simulink model "cccharging"  (R2026a)
settings: Solver=VariableStepAuto  StopTime=3600*nHours
InitFcn:
  | CCCV_parameters
libraries: fl_lib x4, batt_lib x2, nesl_utility x1
settings Model: Creator=clapierr  LastModifiedBy=User
settings SimscapeCC: SimscapeNominalValues="[{\"value\":\"1\",\"unit\":\"A\"},{\"value\":\"1\",\"unit\":\"bar\"},{\"value\":\"1\",\"unit\":\"cm^2\"},{\"value\":\"1\",\"unit\":\"cm^3/s\"},{\"value\":\"1\",\"unit\":\"kJ/kg\"},{\"value\":\"1\",\"unit\":\"kW\"},{\"value\":\"1\",\"unit\":\"l\"},{\"value\":\"1\",\"unit\":\"N\"},{\"value\":\"1\",\"unit\":\"N*m\"},{\"value\":\"1\",\"unit\":\"V\"}]"  SimscapeLogType=none  SimscapeLogDataHistory=5000.0

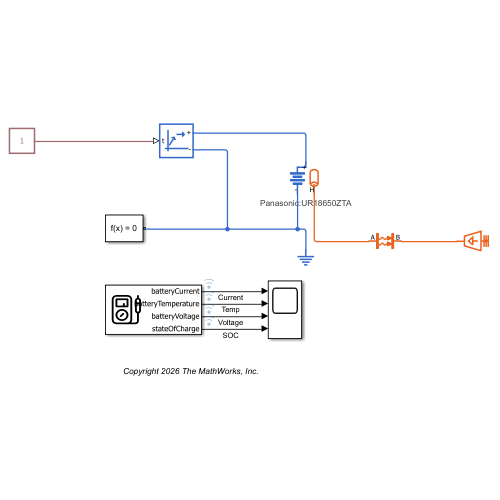
[thumbnail: Simulink's stored preview of the top-level diagram]
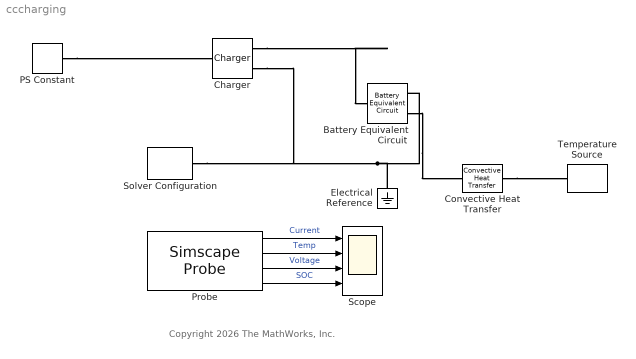
== system cccharging ==
  note: Copyright 2026 The MathWorks, Inc.
  Battery Equivalent Circuit : batt_lib/Cells/Battery Equivalent Circuit  PartSpecification="{\"CollectionId\":\"MW.SimscapeBattery\",\"CollectionVersion\":\"1.0.0\",\"DatasetId\":\"Panasonic|UR18650ZTA|simscape.battery.batteryEquivalentCircuit\",\"DisplayName\":\"Panasonic:UR18650ZTA\"}"  BatteryCapacity=2.65 % Datasheet derived hr*A  ThermalModel=simscape.battery.enum.cells.BatteryThermalModel.LumpedThermalMass  ExtrapolationMethod=simscape.enum.extrapolation.linear  SOCBreakpoints=[0 0.01 0.02 0.03 0.04 0.05 0.06 0.07 0.08 0.09 0.1 0.11 0.12 0.13 0.14 0.15 0.16 0.17 0.18 0.19 0.2 0.21 0.22 0.23 0.24 0.25 0.26 0.27 0.28 0.29 0.3 0.31 0.32 0.33 0.34 0.35 0.36 0.37 0.38 0.39 0.4 0.41 0.42 0.43 0.44 0.45 0.46 0.47 0.48 0.49 0.5 0.51 0.52 0.53 0.54 0.55 0.56 0.57 0.58 0.59 0.6 0.61 0.62 0.63 0.64 0.65 0.66 0.67 0.68 0.69 0.7 0.71 0.72 0.73 0.74 0.75 0.76 0.77 0.78 0.79 0.8 0.81 0.82 0.83 0.84 0.85 0.86 0.87 0.88 0.89 0.9 0.91 0.92 0.93 0.94 0.95 0.96 0.97 0.98 0.99 1] % Datasheet derived  TemperatureBreakpoints=[0 25 40 60] % Datasheet derived degC  OpenCircuitVoltage=[3.04339 3.19969 3.32733 3.41897 3.47789 3.5189 3.54757 3.56926 3.58543 3.59715 3.60656 3.61458 3.62125 3.62859 3.63585 3.64117 3.64677 3.65281 3.65754 3.6622 3.66686 3.67118 3.67547 3.67953 3.68333 3.68679 3.68929 3.69163 3.69398 3.69633 3.69868 3.70108 3.7035 3.70592 3.70834 3.71076 3.71334 3.71599 3.71889 3.72198 3.72508 3.72817 3.73126 3.73436 3.73745 3.74054 3.74364 3.74686 3.75011 3.75346 3.75768 3.7621 3.76652 3.77094 3.77575 3.78058 3.78546 3.79147 3.79777 3.80409 3.8104 3.81672 3.82303 3.82935 3.83618 3.84344 3.8508 3.85816 3.86553 3.87289 3.88052 3.88833 3.89603 3.90423 3.91256 3.92124 3.93029 3.93933 3.94837 3.95788 3.96788 3.97854 3.98931 4.00008 4.01149 4.02304 4.03459 4.04614 4.05768 4.06947 4.08184 4.09422 4.1067 4.11982 4.1326 4.14615 4.15754 4.16699 4.17222 4.18119 4.30838] % Datasheet derived V  OpenCircuitVoltageThermal=[3.04339 3.04339 3.04339 3.04339;3.19969 3.19969 3.19969 3.19969;3.32733 3.32733 3.32733 3.32733;3.41897 3.41897 3.41897 3.41897;3.47789 3.47789 3.47789 3.47789;3.5189 3.5189 3.5189 3.5189;3.54757 3.54757 3.54757 3.54757;3.56926 3.56926 3.56926 3.56926;3.58543 3.58543 3.58543 3.58543;3.59715 3.59715 3.59715 3.59715;3.60656 3.60656 3.60656 3.60656;3.61458 3.61458 3.61458 3.61458;3.62125 3.62125 3.62125 3.62125;3.62859 3.62859 3.62859 3.62859;3.63585 3.63585 3.63585 3.63585;3.64117 3.64117 3.64117 3.64117;3.64677 3.64677 3.64677 3.64677;3.65281 3.65281 3.65281 3.65281;3.65754 3.65754 3.65754 3.65754;3.6622 3.6622 3.6622 3.6622;3.66686 3.66686 3.66686 3.66686;3.67118 3.67118 3.67118 3.67118;3.67547 3.67547 3.67547 3.67547;3.67953 3.67953 3.67953 3.67953;3.68333 3.68333 3.68333 3.68333;3.68679 3.68679 3.68679 3.68679;3.68929 3.68929 3.68929 3.68929;3.69163 3.69163 3.69163 3.69163;3.69398 3.69398 3.69398 3.69398;3.69633 3.69633 3.69633 3.69633;3.69868 3.69868 3.69868 3.69868;3.70108 3.70108 3.70108 3.70108;3.7035 3.7035 3.7035 3.7035;3.70592 3.70592 3.70592 3.70592;3.70834 3.70834 3.70834 3.70834;3.71076 3.71076 3.71076 3.71076;3.71334 3.71334 3.71334 3.71334;3.71599 3.71599 3.71599 3.71599;3.71889 3.71889 3.71889 3.71889;3.72198 3.72198 3.72198 3.72198;3.72508 3.72508 3.72508 3.72508;3.72817 3.72817 3.72817 3.72817;3.73126 3.73126 3.73126 3.73126;3.73436 3.73436 3.73436 3.73436;3.73745 3.73745 3.73745 3.73745;3.74054 3.74054 3.74054 3.74054;3.74364 3.74364 3.74364 3.74364;3.74686 3.74686 3.74686 3.74686;3.75011 3.75011 3.75011 3.75011;3.75346 3.75346 3.75346 3.75346;3.75768 3.75768 3.75768 3.75768;3.7621 3.7621 3.7621 3.7621;3.76652 3.76652 3.76652 3.76652;3.77094 3.77094 3.77094 3.77094;3.77575 3.77575 3.77575 3.77575;3.78058 3.78058 3.78058 3.78058;3.78546 3.78546 3.78546 3.78546;3.79147 3.79147 3.79147 3.79147;3.79777 3.79777 3.79777 3.79777;3.80409 3.80409 3.80409 3.80409;3.8104 3.8104 3.8104 3.8104;3.81672 3.81672 3.81672 3.81672;3.82303 3.82303 3.82303 3.82303;3.82935 3.82935 3.82935 3.82935;3.83618 3.83618 3.83618 3.83618;3.84344 3.84344 3.84344 3.84344;3.8508 3.8508 3.8508 3.8508;3.85816 3.85816 3.85816 3.85816;3.86553 3.86553 3.86553 3.86553;3.87289 3.87289 3.87289 3.87289;3.88052 3.88052 3.88052 3.88052;3.88833 3.88833 3.88833 3.88833;3.89603 3.89603 3.89603 3.89603;3.90423 3.90423 3.90423 3.90423;3.91256 3.91256 3.91256 3.91256;3.92124 3.92124 3.92124 3.92124;3.93029 3.93029 3.93029 3.93029;3.93933 3.93933 3.93933 3.93933;3.94837 3.94837 3.94837 3.94837;3.95788 3.95788 3.95788 3.95788;3.96788 3.96788 3.96788 3.96788;3.97854 3.97854 3.97854 3.97854;3.98931 3.98931 3.98931 3.98931;4.00008 4.00008 4.00008 4.00008;4.01149 4.01149 4.01149 4.01149;4.02304 4.02304 4.02304 4.02304;4.03459 4.03459 4.03459 4.03459;4.04614 4.04614 4.04614 4.04614;4.05768 4.05768 4.05768 4.05768;4.06947 4.06947 4.06947 4.06947;4.08184 4.08184 4.08184 4.08184;4.09422 4.09422 4.09422 4.09422;4.1067 4.1067 4.1067 4.1067;4.11982 4.11982 4.11982 4.11982;4.1326 4.1326 4.1326 4.1326;4.14615 4.14615 4.14615 4.14615;4.15754 4.15754 4.15754 4.15754;4.16699 4.16699 4.16699 4.16699;4.17222 4.17222 4.17222 4.17222;4.18119 4.18119 4.18119 4.18119;4.30838 4.30838 4.30838 4.30838] % Datasheet derived V  VoltageRange=[2.7 Inf] % Datasheet derived V  HysteresisModel=simscape.battery.enum.cells.HysteresisModel.none  MaximumHysteresisVoltage=[0, 0, 0, 0, 0, 0, 0] % Parameter not set V  InstantaneousHysteresisVoltage=[0, 0, 0, 0, 0, 0, 0] % Parameter not set V  HysteresisRate=0.1 % Parameter not set  MaximumHysteresisVoltageThermal=[0, 0, 0; 0, 0, 0; 0, 0, 0; 0, 0, 0; 0, 0, 0; 0, 0, 0; 0, 0, 0] % Parameter not set V  InstantaneousHysteresisVoltageThermal=[0, 0, 0; 0, 0, 0; 0, 0, 0; 0, 0, 0; 0, 0, 0; 0, 0, 0; 0, 0, 0] % Parameter not set V  HysteresisRateThermal=0.1 % Parameter not set  ResistanceSOCBreakpoints=[0 0.01 0.02 0.03 0.04 0.05 0.06 0.07 0.08 0.09 0.1 0.11 0.12 0.13 0.14 0.15 0.16 0.17 0.18 0.19 0.2 0.21 0.22 0.23 0.24 0.25 0.26 0.27 0.28 0.29 0.3 0.31 0.32 0.33 0.34 0.35 0.36 0.37 0.38 0.39 0.4 0.41 0.42 0.43 0.44 0.45 0.46 0.47 0.48 0.49 0.5 0.51 0.52 0.53 0.54 0.55 0.56 0.57 0.58 0.59 0.6 0.61 0.62 0.63 0.64 0.65 0.66 0.67 0.68 0.69 0.7 0.71 0.72 0.73 0.74 0.75 0.76 0.77 0.78 0.79 0.8 0.81 0.82 0.83 0.84 0.85 0.86 0.87 0.88 0.89 0.9 0.91 0.92 0.93 0.94 0.95 0.96 0.97 0.98 0.99 1] % Datasheet derived  ResistanceTemperatureBreakpoints=[0 25 40 60] % Datasheet derived degC  ResistanceCurrentBreakpoints=[-1, 0, 1] % Parameter not set A  CurrentDependence=simscape.battery.enum.cells.CurrentDependence.Disabled  R0=[0.04577 0.0693 0.0871 0.0981 0.10274 0.10473 0.1047 0.10401 0.1029 0.10084 0.09855 0.0961 0.09374 0.0923 0.09098 0.08942 0.08829 0.08779 0.08711 0.08642 0.08573 0.08504 0.08435 0.08362 0.08285 0.0821 0.08136 0.08067 0.07998 0.07929 0.07859 0.07791 0.07723 0.07655 0.07588 0.0752 0.07463 0.07414 0.07372 0.07333 0.07295 0.07256 0.07218 0.07179 0.07141 0.07102 0.07064 0.07034 0.07007 0.06981 0.06973 0.0697 0.06966 0.06963 0.06966 0.06969 0.06974 0.07 0.07016 0.07032 0.07047 0.07062 0.07078 0.07093 0.07117 0.0715 0.07186 0.07221 0.07256 0.07292 0.07332 0.07375 0.0741 0.07448 0.07489 0.07535 0.07584 0.07633 0.07682 0.07759 0.07866 0.07988 0.08112 0.08236 0.08368 0.08499 0.0863 0.08761 0.08891 0.09039 0.09225 0.09411 0.09597 0.09796 0.0995 0.10104 0.10043 0.09826 0.09216 0.08512 0.00997] % Datasheet derived Ohm  R0I=[.0117, .0085, .009; .011, .0085, .009; .0114, .0087, .0092; .0107, .0082, .0088; .0107, .0083, .0091; .0113, .0085, .0089; .0116, .0085, .0089] % Parameter not set Ohm  R0Thermal=[0.10009 0.04577 0.01007 0.01632;0.14613 0.0693 0.01231 0.013;0.1823 0.0871 0.02576 0.02712;0.20605 0.0981 0.03749 0.03657;0.21852 0.10274 0.04624 0.03593;0.22481 0.10473 0.05239 0.04275;0.22685 0.1047 0.05724 0.04532;0.22648 0.10401 0.05969 0.04893;0.22421 0.1029 0.06023 0.05216;0.2204 0.10084 0.06022 0.05386;0.2158 0.09855 0.06061 0.05477;0.21072 0.0961 0.06053 0.05519;0.20518 0.09374 0.05997 0.05515;0.19986 0.0923 0.05976 0.05534;0.19452 0.09098 0.06051 0.05551;0.19005 0.08942 0.06059 0.055;0.18649 0.08829 0.06076 0.05491;0.18308 0.08779 0.06108 0.05531;0.17921 0.08711 0.06095 0.05525;0.17533 0.08642 0.06116 0.05516;0.17188 0.08573 0.06162 0.05537;0.16959 0.08504 0.06197 0.05562;0.16728 0.08435 0.0623 0.05586;0.16489 0.08362 0.06255 0.05603;0.16242 0.08285 0.06272 0.0561;0.15982 0.0821 0.06284 0.05605;0.15726 0.08136 0.06262 0.05568;0.15524 0.08067 0.06235 0.05525;0.15322 0.07998 0.06208 0.05483;0.1512 0.07929 0.06181 0.05441;0.14918 0.07859 0.06154 0.05399;0.14718 0.07791 0.06129 0.05359;0.14518 0.07723 0.06105 0.05316;0.14319 0.07655 0.06062 0.05273;0.14155 0.07588 0.06014 0.0523;0.14028 0.0752 0.05965 0.05186;0.13906 0.07463 0.05921 0.05149;0.13787 0.07414 0.0588 0.05114;0.13676 0.07372 0.05848 0.05087;0.13572 0.07333 0.05823 0.05067;0.13469 0.07295 0.05797 0.05047;0.13365 0.07256 0.05771 0.05028;0.13261 0.07218 0.05746 0.0497;0.13157 0.07179 0.0572 0.04908;0.13053 0.07141 0.05667 0.04845;0.12949 0.07102 0.05603 0.04793;0.1286 0.07064 0.05539 0.04744;0.12808 0.07034 0.05479 0.04699;0.12757 0.07007 0.0542 0.04656;0.1271 0.06981 0.05364 0.04615;0.12693 0.06973 0.05339 0.04605;0.12682 0.0697 0.0532 0.04601;0.12672 0.06966 0.05301 0.04589;0.12661 0.06963 0.05283 0.04564;0.12664 0.06966 0.05277 0.04553;0.12668 0.06969 0.05273 0.04542;0.12673 0.06974 0.0527 0.04507;0.12716 0.07 0.05306 0.04491;0.12758 0.07016 0.053 0.04485;0.128 0.07032 0.0529 0.04479;0.12841 0.07047 0.0528 0.04474;0.12883 0.07062 0.0527 0.04468;0.12925 0.07078 0.05261 0.04463;0.12967 0.07093 0.05251 0.04457;0.13027 0.07117 0.05259 0.04469;0.13101 0.0715 0.05282 0.04497;0.13204 0.07186 0.05308 0.04484;0.13321 0.07221 0.05335 0.04472;0.13439 0.07256 0.0532 0.04459;0.13557 0.07292 0.05301 0.04446;0.13684 0.07332 0.05292 0.04443;0.13817 0.07375 0.05288 0.04428;0.13946 0.0741 0.05281 0.04407;0.14091 0.07448 0.05291 0.04404;0.14233 0.07489 0.05306 0.04405;0.14388 0.07535 0.05333 0.04418;0.14556 0.07584 0.05372 0.04444;0.14723 0.07633 0.05411 0.0447;0.14891 0.07682 0.0545 0.04496;0.15108 0.07759 0.05506 0.04537;0.15372 0.07866 0.05578 0.04596;0.15659 0.07988 0.05673 0.04678;0.1595 0.08112 0.0574 0.04703;0.16241 0.08236 0.05796 0.04728;0.16616 0.08368 0.05874 0.04774;0.17134 0.08499 0.05957 0.04825;0.17651 0.0863 0.0604 0.04877;0.18169 0.08761 0.06123 0.04928;0.18774 0.08891 0.06206 0.04979;0.19646 0.09039 0.06297 0.05038;0.20538 0.09225 0.06408 0.05118;0.2143 0.09411 0.0652 0.05198;0.22836 0.09597 0.06593 0.05281;0.24309 0.09796 0.06644 0.05348;0.25899 0.0995 0.06683 0.05394;0.28056 0.10104 0.06749 0.05466;0.30009 0.10043 0.0674 0.05464;0.31508 0.09826 0.06607 0.05332;0.32861 0.09216 0.06054 0.05002;0.31916 0.08512 0.05631 0.04686;0.33322 0.00997 0.09284 0.03396] % Datasheet derived Ohm  R0ThermalI=repmat([.0117, .0085, .009; .011, .0085, .009; .0114, .0087, .0092; .0107, .0082, .0088; .0107, .0083, .0091; .0113, .0085, .0089; .0116, .0085, .0089], 1, 1, 3) % Parameter not set Ohm  DischargeR0=[.0085, .0085, .0087, .0082, .0083, .0085, .0085] % Parameter not set Ohm  ChargeR0=[.0085, .0085, .0087, .0082, .0083, .0085, .0085] % Parameter not set Ohm  ChargeR0Thermal=[.0117, .0085, .009; .011, .0085, .009; .0114, .0087, .0092; .0107, .0082, .0088; .0107, .0083, .0091; .0113, .0085, .0089; .0116, .0085, .0089] % Parameter not set Ohm  DischargeR0Thermal=[.0117, .0085, .009; .011, .0085, .009; .0114, .0087, .0092; .0107, .0082, .0088; .0107, .0083, .0091; .0113, .0085, .0089; .0116, .0085, .0089] % Parameter not set Ohm  RCPairs=simscape.battery.enum.cells.RCPairs.noDynamics  R1=[.0029, .0024, .0026, .0016, .0023, .0018, .0017] % Parameter not set Ohm  Tau1=[36, 45, 105, 29, 77, 33, 39] % Parameter not set s  R2=[.0029, .0024, .0026, .0016, .0023, .0018, .0017] % Parameter not set Ohm  Tau2=[36, 45, 105, 29, 77, 33, 39] % Parameter not set s  R3=[.0029, .0024, .0026, .0016, .0023, .0018, .0017] % Parameter not set Ohm  Tau3=[36, 45, 105, 29, 77, 33, 39] % Parameter not set s  R1I=[.0109, .0029, .0013; .0069, .0024, .0012; .0047, .0026, .0013; .0034, .0016, .001; .0033, .0023, .0014; .0033, .0018, .0011; .0028, .0017, .0011] % Parameter not set Ohm  Tau1I=[20, 36, 39; 31, 45, 39; 109, 105, 61; 36, 29, 26; 59, 77, 67; 40, 33, 29; 25, 39, 33] % Parameter not set s  R2I=[.0109, .0029, .0013; .0069, .0024, .0012; .0047, .0026, .0013; .0034, .0016, .001; .0033, .0023, .0014; .0033, .0018, .0011; .0028, .0017, .0011] % Parameter not set Ohm  Tau2I=[20, 36, 39; 31, 45, 39; 109, 105, 61; 36, 29, 26; 59, 77, 67; 40, 33, 29; 25, 39, 33] % Parameter not set s  R3I=[.0109, .0029, .0013; .0069, .0024, .0012; .0047, .0026, .0013; .0034, .0016, .001; .0033, .0023, .0014; .0033, .0018, .0011; .0028, .0017, .0011] % Parameter not set Ohm  Tau3I=[20, 36, 39; 31, 45, 39; 109, 105, 61; 36, 29, 26; 59, 77, 67; 40, 33, 29; 25, 39, 33] % Parameter not set s  DischargeR1=[.0029, .0024, .0026, .0016, .0023, .0018, .0017] % Parameter not set Ohm  DischargeTau1=[36, 45, 105, 29, 77, 33, 39] % Parameter not set s  ChargeR1=[.0029, .0024, .0026, .0016, .0023, .0018, .0017] % Parameter not set Ohm  ChargeTau1=[36, 45, 105, 29, 77, 33, 39] % Parameter not set s  DischargeR2=[.0029, .0024, .0026, .0016, .0023, .0018, .0017] % Parameter not set Ohm  DischargeTau2=[36, 45, 105, 29, 77, 33, 39] % Parameter not set s  ChargeR2=[.0029, .0024, .0026, .0016, .0023, .0018, .0017] % Parameter not set Ohm  ChargeTau2=[36, 45, 105, 29, 77, 33, 39] % Parameter not set s  DischargeR3=[.0029, .0024, .0026, .0016, .0023, .0018, .0017] % Parameter not set Ohm  DischargeTau3=[36, 45, 105, 29, 77, 33, 39] % Parameter not set s  ChargeR3=[.0029, .0024, .0026, .0016, .0023, .0018, .0017] % Parameter not set Ohm  ChargeTau3=[36, 45, 105, 29, 77, 33, 39] % Parameter not set s  R1Thermal=[.0109, .0029, .0013; .0069, .0024, .0012; .0047, .0026, .0013; .0034, .0016, .001; .0033, .0023, .0014; .0033, .0018, .0011; .0028, .0017, .0011] % Parameter not set Ohm  Tau1Thermal=[20, 36, 39; 31, 45, 39; 109, 105, 61; 36, 29, 26; 59, 77, 67; 40, 33, 29; 25, 39, 33] % Parameter not set s  R2Thermal=[.0109, .0029, .0013; .0069, .0024, .0012; .0047, .0026, .0013; .0034, .0016, .001; .0033, .0023, .0014; .0033, .0018, .0011; .0028, .0017, .0011] % Parameter not set Ohm  Tau2Thermal=[20, 36, 39; 31, 45, 39; 109, 105, 61; 36, 29, 26; 59, 77, 67; 40, 33, 29; 25, 39, 33] % Parameter not set s  R3Thermal=[.0109, .0029, .0013; .0069, .0024, .0012; .0047, .0026, .0013; .0034, .0016, .001; .0033, .0023, .0014; .0033, .0018, .0011; .0028, .0017, .0011] % Parameter not set Ohm  Tau3Thermal=[20, 36, 39; 31, 45, 39; 109, 105, 61; 36, 29, 26; 59, 77, 67; 40, 33, 29; 25, 39, 33] % Parameter not set s  R1ThermalI=repmat([.0109, .0029, .0013; .0069, .0024, .0012; .0047, .0026, .0013; .0034, .0016, .001; .0033, .0023, .0014; .0033, .0018, .0011; .0028, .0017, .0011], 1, 1, 3) % Parameter not set Ohm  Tau1ThermalI=repmat([20, 36, 39; 31, 45, 39; 109, 105, 61; 36, 29, 26; 59, 77, 67; 40, 33, 29; 25, 39, 33], 1, 1, 3) % Parameter not set s  R2ThermalI=repmat([.0109, .0029, .0013; .0069, .0024, .0012; .0047, .0026, .0013; .0034, .0016, .001; .0033, .0023, .0014; .0033, .0018, .0011; .0028, .0017, .0011], 1, 1, 3) % Parameter not set Ohm  Tau2ThermalI=repmat([20, 36, 39; 31, 45, 39; 109, 105, 61; 36, 29, 26; 59, 77, 67; 40, 33, 29; 25, 39, 33], 1, 1, 3) % Parameter not set s  R3ThermalI=repmat([.0109, .0029, .0013; .0069, .0024, .0012; .0047, .0026, .0013; .0034, .0016, .001; .0033, .0023, .0014; .0033, .0018, .0011; .0028, .0017, .0011], 1, 1, 3) % Parameter not set Ohm  Tau3ThermalI=repmat([20, 36, 39; 31, 45, 39; 109, 105, 61; 36, 29, 26; 59, 77, 67; 40, 33, 29; 25, 39, 33], 1, 1, 3) % Parameter not set s  DischargeR1Thermal=[.0109, .0029, .0013; .0069, .0024, .0012; .0047, .0026, .0013; .0034, .0016, .001; .0033, .0023, .0014; .0033, .0018, .0011; .0028, .0017, .0011] % Parameter not set Ohm  DischargeTau1Thermal=[20, 36, 39; 31, 45, 39; 109, 105, 61; 36, 29, 26; 59, 77, 67; 40, 33, 29; 25, 39, 33] % Parameter not set s  ChargeR1Thermal=[.0109, .0029, .0013; .0069, .0024, .0012; .0047, .0026, .0013; .0034, .0016, .001; .0033, .0023, .0014; .0033, .0018, .0011; .0028, .0017, .0011] % Parameter not set Ohm  ChargeTau1Thermal=[20, 36, 39; 31, 45, 39; 109, 105, 61; 36, 29, 26; 59, 77, 67; 40, 33, 29; 25, 39, 33] % Parameter not set s  DischargeR2Thermal=[.0109, .0029, .0013; .0069, .0024, .0012; .0047, .0026, .0013; .0034, .0016, .001; .0033, .0023, .0014; .0033, .0018, .0011; .0028, .0017, .0011] % Parameter not set Ohm  DischargeTau2Thermal=[20, 36, 39; 31, 45, 39; 109, 105, 61; 36, 29, 26; 59, 77, 67; 40, 33, 29; 25, 39, 33] % Parameter not set s  ChargeR2Thermal=[.0109, .0029, .0013; .0069, .0024, .0012; .0047, .0026, .0013; .0034, .0016, .001; .0033, .0023, .0014; .0033, .0018, .0011; .0028, .0017, .0011] % Parameter not set Ohm  ChargeTau2Thermal=[20, 36, 39; 31, 45, 39; 109, 105, 61; 36, 29, 26; 59, 77, 67; 40, 33, 29; 25, 39, 33] % Parameter not set s  DischargeR3Thermal=[.0109, .0029, .0013; .0069, .0024, .0012; .0047, .0026, .0013; .0034, .0016, .001; .0033, .0023, .0014; .0033, .0018, .0011; .0028, .0017, .0011] % Parameter not set Ohm  DischargeTau3Thermal=[20, 36, 39; 31, 45, 39; 109, 105, 61; 36, 29, 26; 59, 77, 67; 40, 33, 29; 25, 39, 33] % Parameter not set s  ChargeR3Thermal=[.0109, .0029, .0013; .0069, .0024, .0012; .0047, .0026, .0013; .0034, .0016, .001; .0033, .0023, .0014; .0033, .0018, .0011; .0028, .0017, .0011] % Parameter not set Ohm  ChargeTau3Thermal=[20, 36, 39; 31, 45, 39; 109, 105, 61; 36, 29, 26; 59, 77, 67; 40, 33, 29; 25, 39, 33] % Parameter not set s  SelfDischargeResistor=simscape.battery.enum.cells.BatteryEnable.Disabled  SelfDischargeR=7e3 % Parameter not set Ohm  SelfDischargeRThermal=[8000, 7000, 6000] % Parameter not set Ohm  CyclingAgingMethod=simscape.battery.enum.cells.CyclingAgingMethod.tableN  CycleCalculationMethod=simscape.battery.enum.cells.CycleCalculationMethod.EquivalentCycles  NumDisCycles=100 % Parameter not set  OCVChange=0 % Parameter not set  R0Change=0 % Parameter not set  CapacityChange=0 % Parameter not set  SelfDischargeRChange=0 % Parameter not set  R1Change=0 % Parameter not set  R2Change=0 % Parameter not set  R3Change=0 % Parameter not set  NumDisCyclesBreakpoints=[0 7 13 19 25 31 37 43 49 55 61 67 73 79 85 91 97 103 109 115 121 127 133 139 145 151 157 163 169 175 181 187 193 199 205 211 217 223 229 235 241 247 253 259 265 271 277 283 289 295 301 307 313 319 325 331 337 343 349 355 361 367 373 379 385 391 397 403 409 415 421 427 433 439 445 451 457 463 469 475 481 487 493 499] % Datasheet derived  AgingTemperatureBreakpoints=[298.15, 323.15] % Parameter not set K  AgingCurrentBreakpoints=[-.1, -.5, -5] % Parameter not set A  OCVChangeVec=[0 -1.7373 -2.9889 -3.1115 -3.2033 -3.2746 -3.3973 -3.5142 -3.6524 -3.7953 -3.9595 -4.1213 -4.2764 -4.433 -4.5902 -4.7179 -4.8412 -4.9645 -5.0868 -5.209 -5.3312 -5.4534 -5.5742 -5.6906 -5.807 -5.9213 -6.0353 -6.1494 -6.2635 -6.3776 -6.4816 -6.5242 -6.5668 -6.6094 -6.6519 -6.6945 -6.7371 -6.7797 -6.8223 -6.8649 -6.9072 -6.9493 -6.9914 -7.0334 -7.0755 -7.1175 -7.1552 -7.187 -7.2188 -7.2507 -7.2825 -7.3143 -7.3461 -7.3779 -7.4097 -7.4415 -7.4714 -7.4908 -7.5103 -7.5297 -7.5491 -7.5685 -7.588 -7.6074 -7.6268 -7.6463 -7.6656 -7.6848 -7.7105 -7.7394 -7.7683 -7.7971 -7.826 -7.8549 -7.8838 -7.9121 -7.9392 -7.9554 -7.9697 -7.9841 -7.9984 -8.0127 -8.0271 -8.0414] % Datasheet derived  OCVChangeThermal=[0, 0; 0, 0; 0, 0; 0, 0] % Parameter not set  R0ChangeVec=[0 0 0 0 0 0 0 0 0 0 0 0 0 0 0 0 0 0 0 0 0 0 0 0 0 0 0 0 0 0 0 0 0 0 0 0 0 0 0 0 0 0 0 0 0 0 0 0 0 0 0 0 0 0 0 0 0 0 0 0 0 0 0 0 0 0 0 0 0 0 0 0 0 0 0 0 0 0 0 0 0 0 0 0] % Parameter assumed  R0ChangeThermal=[0, 0; 0, 0; 0, 0; 0, 0] % Parameter not set  R0ChangeThermalI=repmat(0, 4, 2, 3) % Parameter not set  R0CyclingChangeInitialTarget=0 % Parameter not set  CapacityChangeVec=[0 -0.588 -1.177 -1.765 -2.354 -2.942 -3.527 -4.05 -4.572 -5.095 -5.617 -6.14 -6.662 -7.185 -7.701 -8.127 -8.553 -8.978 -9.404 -9.829 -10.255 -10.68 -11.106 -11.532 -11.957 -12.383 -12.808 -13.234 -13.659 -14.085 -14.473 -14.632 -14.791 -14.95 -15.109 -15.267 -15.426 -15.585 -15.744 -15.903 -16.062 -16.221 -16.379 -16.538 -16.697 -16.856 -16.998 -17.125 -17.253 -17.38 -17.507 -17.634 -17.762 -17.889 -18.016 -18.143 -18.263 -18.341 -18.418 -18.496 -18.574 -18.651 -18.729 -18.807 -18.885 -18.962 -19.04 -19.118 -19.221 -19.338 -19.455 -19.572 -19.688 -19.805 -19.922 -20.039 -20.156 -20.225 -20.287 -20.349 -20.41 -20.472 -20.534 -20.596] % Datasheet derived  CapacityChangeThermal=[0, 0; 0, 0; 0, 0; 0, 0] % Parameter not set  CapacityChangeThermalI=repmat(0, 4, 2, 3) % Parameter not set  CapacityCyclingChangeInitialTarget=0 % Parameter not set  SelfDischargeRChangeVec=[0, 0, 0, 0] % Parameter not set  SelfDischargeRChangeThermal=[0, 0; 0, 0; 0, 0; 0, 0] % Parameter not set  SelfDischargeRChangeThermalI=repmat(0, 4, 2, 3) % Parameter not set  SelfDischargeRCyclingChangeInitialTarget=0 % Parameter not set  R1ChangeVec=[0, 0, 0, 0] % Parameter not set  R1ChangeThermal=[0, 0; 0, 0; 0, 0; 0, 0] % Parameter not set  R1ChangeThermalI=repmat(0, 4, 2, 3) % Parameter not set  R1CyclingChangeInitialTarget=0 % Parameter not set  R2ChangeVec=[0, 0, 0, 0] % Parameter not set  R2ChangeThermal=[0, 0; 0, 0; 0, 0; 0, 0] % Parameter not set  R2ChangeThermalI=repmat(0, 4, 2, 3) % Parameter not set  R2CyclingChangeInitialTarget=0 % Parameter not set  R3ChangeVec=[0, 0, 0, 0] % Parameter not set  R3ChangeThermal=[0, 0; 0, 0; 0, 0; 0, 0] % Parameter not set  R3ChangeThermalI=repmat(0, 4, 2, 3) % Parameter not set  R3CyclingChangeInitialTarget=0 % Parameter not set  CalendarAgeResistance=simscape.battery.enum.cells.BatteryEnable.Disabled  CalendarAgeCapacity=simscape.battery.enum.cells.BatteryEnable.Disabled  CalendarAgingMethod=simscape.battery.enum.cells.CalendarAgingMethod.equation  StorageVariable=simscape.battery.enum.cells.StorageVariable.OCV  OCVDuringStorage=0.9 % Parameter not set  SOCDuringStorage=0.6 % Parameter not set  StorageTimeIntervals=[0] % Parameter not set d  StorageTemperatures=[273] % Parameter not set K  ResistanceScalingOCV=2.2134e6 % Parameter not set  ResistanceScalingOCVOffset=1.632e6 % Parameter not set  ResistanceExponentialIncrease=0.515833569 % Parameter not set V  ResistanceTimeExponent=0.75 % Parameter not set  ResistanceAgeTemperatureBreakpoints=[273.15, 298.15, 323.15] % Parameter not set K  ResistanceAgeTimeBreakpoints=[0, 90, 180, 270] % Parameter not set d  PercentResistanceChange=[0, 0, 0] % Parameter not set  ResistanceTimeBreakpoints=100 % Parameter not set d  PercentResistanceChangeThermal=[0, 0, 0; 0, 0, 0; 0, 0, 0; 0, 0, 0] % Parameter not set  CapacityScalingOCV=1.5097e07 % Parameter not set  CapacityScalingOCVOffset=8.3625e06 % Parameter not set  CapacityExponentialIncrease=0.6011 % Parameter not set V  CapacityTimeExponent=0.75 % Parameter not set  CapacityAgeTemperatureBreakpoints=[273.15, 298.15, 323.15] % Parameter not set K  CapacityAgeTimeBreakpoints=[0, 90, 180, 270] % Parameter not set d  PercentCapacityChange=[0, 0, 0] % Parameter not set  CapacityTimeBreakpoints=100 % Parameter not set d  PercentCapacityChangeThermal=[0, 0, 0; 0, 0, 0; 0, 0, 0; 0, 0, 0] % Parameter not set  SimulationTemperature=298.15 % Parameter not set K  BatteryThermalMass=44.1 % Parameter assumed J/K  NumThermalModels=6 % Parameter not set  ThermalConductivityZ=18 % Parameter not set W/(K*m)  CrossSectionalAreaXY=0.000261 m^2  Height=0.0651 m  ReversibleHeatModel=simscape.battery.enum.cells.ReversibleHeatModel.Disabled  EntropicCoefficient=[0, 0, 0, 0, 0, 0, 0] % Parameter not set mV/K  CurrentDirectionality=simscape.battery.enum.cells.BatteryEnable.Disabled  stateOfCharge_specify=on  stateOfCharge_priority=High  stateOfCharge=0  stateOfCharge_nominal_specify=off  stateOfCharge_nominal_value=1  stateOfCharge_nominal_unit=1  batteryVoltage_specify=off  batteryVoltage_priority=None  batteryVoltage=0 V  batteryVoltage_nominal_specify=off  batteryVoltage_nominal_value=1  batteryVoltage_nominal_unit=V  batteryCurrent_specify=off  batteryCurrent_priority=None  batteryCurrent=0 A  batteryCurrent_nominal_specify=off  batteryCurrent_nominal_value=1  batteryCurrent_nominal_unit=A  numCycles_specify=off  numCycles_priority=High  numCycles=0  numCycles_nominal_specify=off  numCycles_nominal_value=1  numCycles_nominal_unit=1  batteryTemperature_specify=on  batteryTemperature_priority=High  batteryTemperature=AmbientTemp degC  batteryTemperature_nominal_specify=off  batteryTemperature_nominal_value=1  batteryTemperature_nominal_unit=K  hysteresisState_specify=off  hysteresisState_priority=High  hysteresisState=0  hysteresisState_nominal_specify=off  hysteresisState_nominal_value=1  hysteresisState_nominal_unit=1  isExothermFaulted_specify=off  isExothermFaulted_priority=None  isExothermFaulted=0  isExothermFaulted_nominal_specify=off  isExothermFaulted_nominal_value=1  isExothermFaulted_nominal_unit=1  reactionHeatRate_specify=off  reactionHeatRate_priority=None  reactionHeatRate=0 W  reactionHeatRate_nominal_specify=off  reactionHeatRate_nominal_value=1  reactionHeatRate_nominal_unit=W  reactionExtent_specify=off  reactionExtent_priority=None  reactionExtent=0  reactionExtent_nominal_specify=off  reactionExtent_nominal_value=1  reactionExtent_nominal_unit=1
      settings: AttributesFormatString=Panasonic:UR18650ZTA
  Charger : batt_lib/Cyclers/Charger  charging_current=Ccharge A  voltage_threshold=Vthresh V  charging_voltage=Vcharge V  current_threshold=Ccutoff A
  Convective Heat Transfer : fl_lib/Thermal/Thermal Elements/Convective Heat Transfer  thermal_type=foundation.enum.constant_variable.constant  area=SurfaceArea m^2  heat_tr_coeff=20 W/(K*m^2)  min_heat_tr_coeff=1e-3 W/(K*m^2)  T_specify=off  T_priority=None  T=0 K  T_nominal_specify=off  T_nominal_value=1  T_nominal_unit=K  Q_specify=off  Q_priority=None  Q=0 W  Q_nominal_specify=off  Q_nominal_value=1  Q_nominal_unit=W
  Electrical Reference : fl_lib/Electrical/Electrical Elements/Electrical Reference
  PS Constant : fl_lib/Physical Signals/Sources/PS Constant  constant=1
  Probe : SimscapeProbe  BoundBlock=11  Variables="{\"batteryCurrent\":{\"Probing\":\"ON\"},\"batteryTemperature\":{\"Probing\":\"ON\"},\"batteryVoltage\":{\"Probing\":\"ON\"},\"stateOfCharge\":{\"Probing\":\"ON\"}}"
  Scope : Scope  NumInputPorts=4
      settings: ActiveDisplayYMinimum=-0.33124999999999993  ActiveDisplayYMaximum=2.9812499999999997
  Solver Configuration : nesl_utility/Solver Configuration  PhysicalDomain=network_engine_domain  SubClassName=solver  LeftPortType=input  RightPortType=generic  Tones=[]  Harmonics=[]  SimulateNoise=off  Profile=off  UseLocalSampling=off  EnableSwitchedLinearOptims=on  FrequencyDomain=off  UseCCode=off  RelTol=0.001  AbsTol=0.001  MinStep=1e-09  ToWorkspace=off  RevertToSquareIcSolve=off  NumHomotopyIterations=100  PhasorMode=off  PhasorModeNumHarmonics=1  ConsistencySolver=NEWTON_XTOL_AFTER_FTOL  CanonicalOrdering=UNORDERED  OptimizeIntermediates=UNOPTIMIZED  IndexReductionMethod=DerivativeReplacement  DoDC=off  ResidualTolerance=1e-09  ConsistencyTolSource=GLOBAL  ConsistencyAbsTol=0.001  ConsistencyRelTol=0.001  ConsistencyTolFactor=0.001  UseLocalSolver=off  LocalSolverChoice=NE_BACKWARD_EULER_ADVANCER  ResolveIndetEquations=on  FunctionEvalNumThread=1  LocalSolverSampleTime=0.001  DoFixedCost=off  MaxNonlinIter=3  MaxModeIter=2  ComputeImpulses=off  ImpulseIterations=2  LinearAlgebra=auto  LinearAlgebraNumThread=0  EquationFormulation=NE_TIME_EF  DelaysMemoryBudget=1024  AutomaticFiltering=on  FilteringTimeConstant=0.001  PartitionStorageMethod=AS_NEEDED  PartitionMemoryBudget=1024  PartitionMethod=ROBUST  MultibodyUseLocalSolver=off  MultibodyLocalSolverChoice=ODE1  MultibodyLocalSolverSampleTime=0.001
  Temperature Source : fl_lib/Thermal/Thermal Sources/Temperature Source  temperature=AmbientTemp degC
  wires:
  Probe/1 -> Scope/1  "Current"
  Probe/2 -> Scope/2  "Temp"
  Probe/3 -> Scope/3  "Voltage"
  Probe/4 -> Scope/4  "SOC"
  connections:
  Electrical Reference/LConn1 -- Charger/RConn2 -- Solver Configuration/RConn1 -- Battery Equivalent Circuit/RConn1
  Charger/RConn1 -- Battery Equivalent Circuit/LConn1
  PS Constant/RConn1 -- Charger/LConn1
  Battery Equivalent Circuit/RConn2 -- Convective Heat Transfer/LConn1
  Convective Heat Transfer/RConn1 -- Temperature Source/LConn1
